simulink model "task_4_simulink"  (R2020a)
settings: Solver=VariableStepAuto  StartTime=0.0  StopTime=10.0  RelTol=1e-3
settings Model: Creator=sergo  LastModifiedBy=sergo

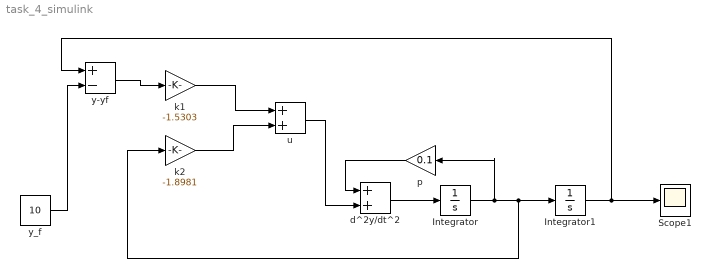
== system task_4_simulink ==
  Integrator : Integrator
  Integrator1 : Integrator
  Scope1 : Scope
  d^2y/dt^2 : Sum
  k1 : Gain  Gain=-1.5303
  k2 : Gain  Gain=-1.8981
  p : Gain  Gain=0.1
  u : Sum
  y-yf : Sum  Inputs=+-
  y_f : Constant  Value=10
  wires:
  d^2y/dt^2/1 -> Integrator/1
  Integrator1/1 -> y-yf/1, Scope1/1
  Integrator/1 -> p/1, k2/1, Integrator1/1
  y_f/1 -> y-yf/2
  y-yf/1 -> k1/1
  k1/1 -> u/1
  k2/1 -> u/2
  p/1 -> d^2y/dt^2/1
  u/1 -> d^2y/dt^2/2
